simulink model "rate_out_of_bounds"  (R2017a)
settings: Solver=VariableStepAuto  StartTime=0.0  StopTime=10.0  RelTol=1e-3
settings Model: Creator=joaomanito  LastModifiedBy=joaomanito

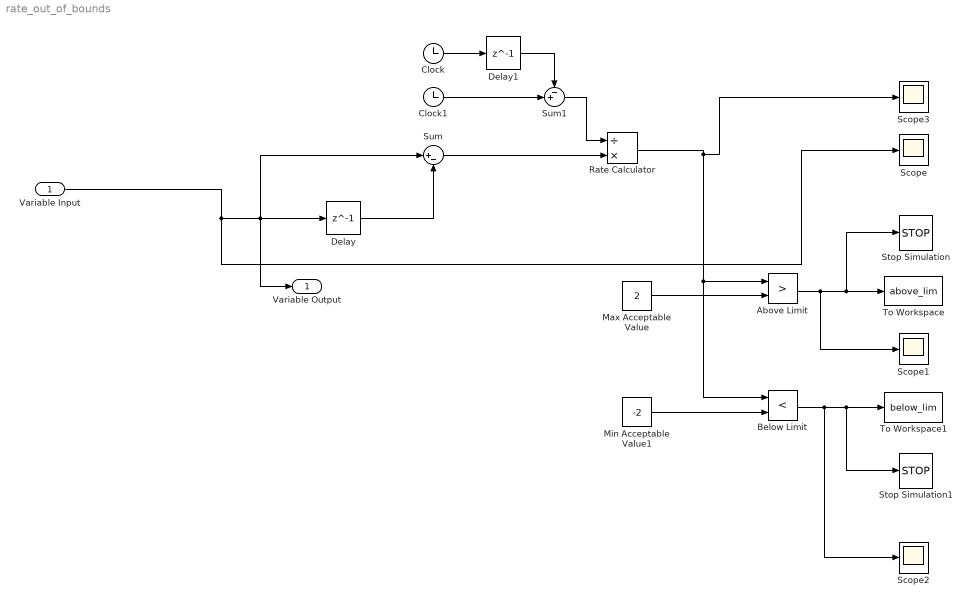
== system rate_out_of_bounds ==
  Variable Input : Inport
  Above Limit : RelationalOperator  Operator=>  OutDataTypeStr=boolean  ZeroCross=off  RndMeth=Simplest
  Below Limit : RelationalOperator  Operator=<  OutDataTypeStr=boolean  ZeroCross=off  RndMeth=Simplest
  Clock : Clock
  Clock1 : Clock
  Delay : Delay  DelayLength=1
  Delay1 : Delay  DelayLength=1
  Max Acceptable Value : Constant  Value=2
  Min Acceptable Value1 : Constant  Value=-2
  Rate Calculator : Product  Inputs=/*
  Scope{,1..3} (4 alike) : Scope
  Stop Simulation : Stop
  Stop Simulation1 : Stop
  Sum : Sum  Inputs=|+-
  Sum1 : Sum  Inputs=-+|
  To Workspace : ToWorkspace  VariableName=above_lim  SaveFormat=Timeseries  SampleTime=-1
      settings: MaxDataPoints=1
  To Workspace1 : ToWorkspace  VariableName=below_lim  SaveFormat=Timeseries  SampleTime=-1
  Variable Output : Outport
  wires:
  Below Limit/1 -> Scope2/1, Stop Simulation1/1, To Workspace1/1
  Above Limit/1 -> Scope1/1, Stop Simulation/1, To Workspace/1
  Variable Input/1 -> Scope/1, Delay/1, Sum/1, Variable Output/1
  Delay/1 -> Sum/2
  Clock/1 -> Delay1/1
  Delay1/1 -> Sum1/1
  Clock1/1 -> Sum1/2
  Sum1/1 -> Rate Calculator/1
  Sum/1 -> Rate Calculator/2
  Rate Calculator/1 -> Scope3/1, Above Limit/1, Below Limit/1
  Min Acceptable Value1/1 -> Below Limit/2
  Max Acceptable Value/1 -> Above Limit/2
